simulink model "BlockControllerPIDSwitchSpeedgoat"  (Simulink 8.8)
settings: configuration reference "WheelSimConfiguration" (kept outside this file)
undefined symbols (not defined in the file): simulator
libraries: simulink x1, dspstat3 x1, simulink_extras x1
settings Model: Creator=At  LastModifiedBy=User  SimulationMode=external
settings ConfigSet: SourceLocation=Base Workspace

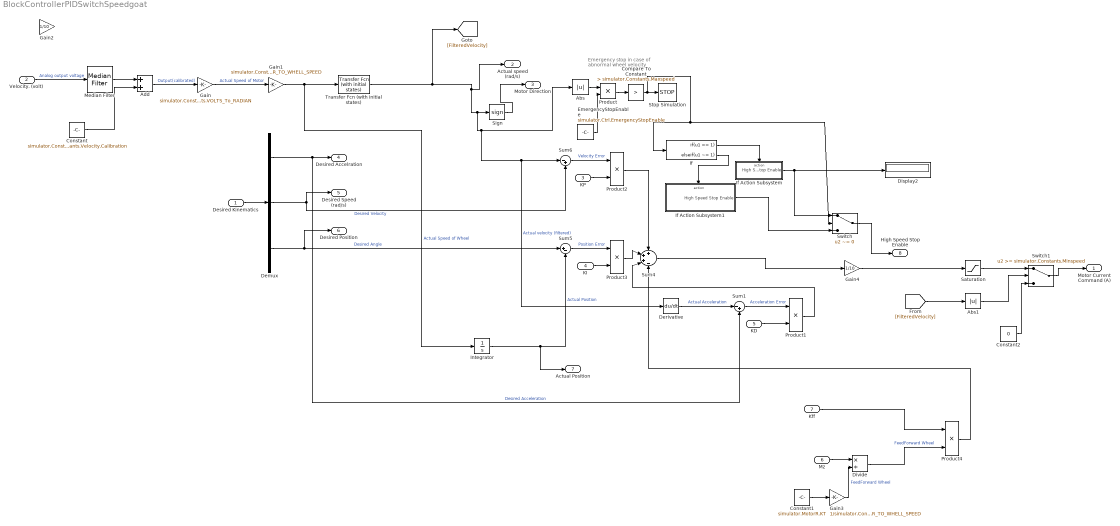
== system BlockControllerPIDSwitchSpeedgoat ==
  note: Emergency stop in case of
      | abnormal wheel velocity
  Desired Kinematics : Inport
  Velocity. (volt) : Inport  Port=2
  KP : Inport  Port=3
  KI : Inport  Port=4
  KD : Inport  Port=5
  Mz : Inport  Port=6
  Kff : Inport  Port=7
  Abs : Abs
  Abs1 : Abs
  Add : Sum
  Compare To Constant : simulink/Logic and Bit Operations/Compare To Constant  relop=>  const=simulator.Constants.Maxspeed  OutDataTypeStr=boolean
  Constant : Constant  Value=simulator.Constants.Velocity.Calibration
  Constant1 : Constant  Value=simulator.MotorR.KT
  Constant2 : Constant  Value=0
  Demux : Demux  Outputs=3
  Derivative : Derivative
  Display2 : Display
  Divide : Product  Inputs=*/
  EmergencyStopEnable : Constant  Value=simulator.Ctrl.EmergencyStopEnable
  Gain : Gain  Gain=simulator.Constants.VOLTS_To_RADIAN
  Gain1 : Gain  Gain=simulator.Constants.MOTOR_TO_WHELL_SPEED
  Gain2 : Gain  Gain=1/10
  Gain3 : Gain  Gain=1/simulator.Constants.MOTOR_TO_WHELL_SPEED
  Gain4 : Gain  Gain=1/10
  If : If  IfExpression=u1 == 1  ElseIfExpressions=u1 ~= 1  ShowElse=off
  If Action Subsystem : Subsystem  TreatAsAtomicUnit=on
  If Action Subsystem1 : Subsystem  TreatAsAtomicUnit=on
  Integrator : Integrator
  Median Filter : dspstat3/Median Filter  WindowLength=3  SimulateUsing=Interpreted execution
  Product{,1..4} (5 alike) : Product  RndMeth=Zero
  Saturation : Saturate  UpperLimit=5  LowerLimit=-5
  Sign : Signum
  Stop Simulation : Stop
  Sum1 : Sum  Inputs=|-+
  Sum4 : Sum  Inputs=+++-
  Sum5 : Sum  Inputs=|+-
  Sum6 : Sum  Inputs=|-+
  Switch : Switch  Criteria=u2 ~= 0
  Switch1 : Switch  Threshold=simulator.Constants.Minspeed
  Transfer Fcn (with initial states) : simulink_extras/Additional Linear/Transfer Fcn (with initial states)  N=simulator.Velocityfilter.num  D=simulator.Velocityfilter.den  X0=0
  Motor Current Command (A) : Outport
  Actual speed (rad/s) : Outport  Port=2
  Motor Direction : Outport  Port=3
  Desired Accelration : Outport  Port=4
  Desired Speed (rad/s) : Outport  Port=5
  Desired Position : Outport  Port=6
  Actual Position : Outport  Port=7  SignalName=Actual Position
  High Speed Stop Enable : Outport  Port=8
  wires:
  Product3/1 -> Sum4/2
  EmergencyStopEnable/1 -> Product/2
  Sum5/1 -> Product3/1  "Position Error"
  Sum6/1 -> Product2/1  "Velocity Error"
  KP/1 -> Product2/2
  Product/1 -> Compare To Constant/1
  Demux/3 -> Desired Position/1, Sum5/1  "Desired Angle"
  Demux/2 -> Sum6/2, Desired Speed (rad/s)/1  "Desired Velocity"
  Desired Kinematics/1 -> Demux/1
  Integrator/1 -> Actual Position/1, Sum5/2  "Actual Position"
  Sign/1 -> Motor Direction/1
  KI/1 -> Product3/2
  Sum4/1 -> Gain4/1
  Abs/1 -> Product/1
  Product2/1 -> Sum4/1
  Gain/1 -> Gain1/1  "Actual Speed of Motor"
  Gain1/1 -> Integrator/1, Transfer Fcn (with initial states)/1  "Actual Speed of Wheel"
  If/1 -> If Action Subsystem/Action
  Compare To Constant/1 -> If/1, Switch/2, Stop Simulation/1
  If/2 -> If Action Subsystem1/Action
  If Action Subsystem/1(High Speed Stop Enable) -> Switch/1, Display2/1
  Switch/1 -> High Speed Stop Enable/1
  If Action Subsystem1/1(High Speed Stop Enable) -> Switch/3
  Demux/1 -> Sum1/2, Desired Accelration/1  "Desired Acceleration"
  Product1/1 -> Sum4/3
  KD/1 -> Product1/2
  Sum1/1 -> Product1/1  "Acceleration Error"
  Derivative/1 -> Sum1/1  "Actual Acceleration"
  Transfer Fcn (with initial states)/1 -> [FilteredVelocity], Derivative/1, Sum6/1, Abs/1, Sign/1, Actual speed (rad/s)/1  "Actual velocity (filtered)"
  Mz/1 -> Divide/1
  Constant1/1 -> Gain3/1
  Gain3/1 -> Divide/2  "FeedForward Wheel"
  Kff/1 -> Product4/1
  Divide/1 -> Product4/2  "FeedForward Wheel"
  Product4/1 -> Sum4/4
  Constant/1 -> Add/2
  Velocity. (volt)/1 -> Median Filter/1  "Analog output voltage"
  Add/1 -> Gain/1  "Output(calibrated)"
  Median Filter/1 -> Add/1
  Switch1/1 -> Motor Current Command (A)/1
  Saturation/1 -> Switch1/1
  [FilteredVelocity] -> Abs1/1
  Constant2/1 -> Switch1/3
  Abs1/1 -> Switch1/2
  Gain4/1 -> Saturation/1

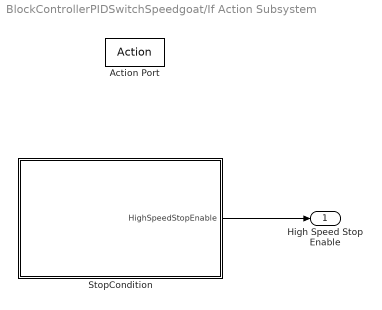
== system BlockControllerPIDSwitchSpeedgoat/If Action Subsystem ==
  Action Port : ActionPort
  StopCondition : MATLAB Function  TreatAsAtomicUnit=on
  High Speed Stop Enable : Outport
  wires:
  StopCondition/1(HighSpeedStopEnable) -> High Speed Stop Enable/1

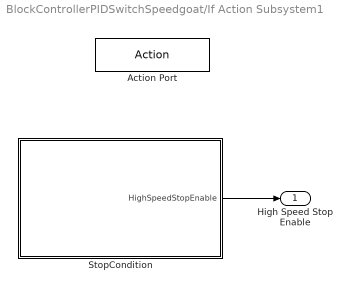
== system BlockControllerPIDSwitchSpeedgoat/If Action Subsystem1 ==
  Action Port : ActionPort
  StopCondition : MATLAB Function  TreatAsAtomicUnit=on
  High Speed Stop Enable : Outport
  wires:
  StopCondition/1(HighSpeedStopEnable) -> High Speed Stop Enable/1

== matlab function If Action Subsystem1/StopCondition ==
  data: HighSpeedStopEnable output double
function HighSpeedStopEnable   = stopcondition(  )

%% This function determines the reason for stoping the system


    
HighSpeedStopEnable=0;

== matlab function If Action Subsystem/StopCondition ==
  data: HighSpeedStopEnable output double
function HighSpeedStopEnable   = stopcondition(  )

%% This function determines the reason for stoping the system


    
HighSpeedStopEnable=1;
